simulink library "dspstat3"  (Simulink 8.0)
settings: Solver=ode45  SolverMode=SingleTasking  StartTime=0.0  StopTime=10.0  RelTol=1e-3
values from neighbouring files (symbols this model uses):
  D = D + B    [rebuffer_delay.m]
undefined symbols (not defined in the file or in its folder): Floor, Rows
libraries: dspsigattribs x3, dspsigops x1, dspindex x1, dspobslib x1, dspstat3 x1
settings Model: RequirementInfo=9  Creator=szlotkin  LastModifiedBy=lij  CovMetricSettings=d  ExtModeAutoUpdateStatusClock=off

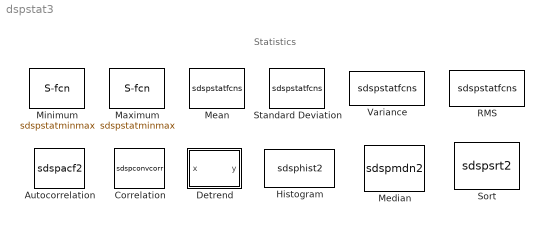
== system dspstat3 ==
  note: Statistics
  Autocorrelation : S-Function  DialogController=dspDDGCreate  DialogControllerArgs=DataTag0  FunctionName=sdspacf2  Parameters=AllPositiveLags,maxlag,bias,domain,outputMin,outputMax,dtInfo.prodOutputMode,dtInfo.prodOutputWordLength,dtInfo.prodOutputFracLength,dtInfo.accumMode,dtInfo.accumWordLength,dtInfo.accumFracLength,dtInfo.outputMode,dtInfo.outputWordLength,dtInfo.outputFracLength,dtInfo.roundingMode,dtInfo.overflowMode  EnableBusSupport=off  mask(Autocorrelation){AllPositiveLags=on, maxlag=1, bias=None, domain=Time, additionalParams=off, allowOverrides=on, outputMode=Same as accumulator, outputWordLength=16, outputFracLength=15, outputDataTypeStr=Inherit: Same as accumulator, outputLastDataTypeStr=Inherit: Same as accumulator, outputMin=[], outputMax=[], accumMode=Inherit via internal rule, accumWordLength=32, accumFracLength=30, accumDataTypeStr=Inherit: Inherit via internal rule, accumLastDataTypeStr=Inherit: Inherit via internal rule, prodOutputMode=Inherit via internal rule, prodOutputWordLength=32, prodOutputFracLength=30, prodOutputDataTypeStr=Inherit: Inherit via internal rule, prodOutputLastDataTypeStr=Inherit: Inherit via internal rule, roundingMode=Floor, overflowMode=off, LockScale=off}
      mask prompts: AllPositiveLags "Compute all non-negative lags"; maxlag "Maximum non-negative lag (less than input length):"; bias "Scaling:"; domain "Computation domain:"; additionalParams "--------------- Show additional parameters ---------------"; allowOverrides "Allow overrides from DSP Fixed-Point Attributes blocks"; outputMode "Fixed-point output attributes:"; outputWordLength "Output word length:"; outputFracLength "Output fraction length:"; outputDataTypeStr "Output data type string:"; outputLastDataTypeStr "Last output data type string:"; outputMin "Output minimum:"; outputMax "Output maximum:"; accumMode "Fixed-point accumulator attributes:"; accumWordLength "Accumulator word length:"; accumFracLength "Accumulator fraction length:"; accumDataTypeStr "Accum data type string:"; accumLastDataTypeStr "Last accum data type string:"; prodOutputMode "Fixed-point product output attributes:"; prodOutputWordLength "Product output word length:"; prodOutputFracLength "Product output fraction length:"; prodOutputDataTypeStr "ProdOutput data type string:"; prodOutputLastDataTypeStr "Last prodOutput data type string:"; roundingMode "Round integer calculations toward:"; overflowMode "Saturate on integer overflow"; LockScale "Lock scaling"
      mask help: Compute the autocorrelation along the first dimension of an N-D input array.
      mask init:
      | blkh   = gcbh;
      | dtRows = dspblkGetAutocorrelationDTRowInfo();
      | dtInfo = dspGetUDTFixptDataTypeInfo(blkh, dtRows, true);
      mask Help: eval('blocksethelp');
      mask StyleString: checkbox,edit,popup(None|Biased|Unbiased|Unity at zero-lag),popup(Time|Frequency),checkbox,checkbox,popup(Same as accumulator|Same as product output|Same as input|Binary point scaling|Slope and bias scaling|User-defined),edit,edit,unidt({a=10|12|13|}{i=Inherit: Same as input|Inherit: Same as product output|Inherit: Same as accumulator}{s=UDTBinaryPointMode}{g=UDTInheritSign}),edit,min,max,popup(Inherit via internal rule|Same as product output|Same as input|Binary point scaling|Slope and bias scaling|User-defined),edit,edit,unidt({a=17|||}{i=Inherit: Inherit via internal rule|Inherit: Same as input|Inherit: Same as product output}{s=UDTBinaryPointMode}{g=UDTInheritSign}),edit,popup(Inherit via internal rule|Same as input|Binary point scaling|Slope and bias scaling|User-defined),edit,edit,unidt({a=22|||}{i=Inherit: Inherit via internal rule|Inherit: Same as input}{s=UDTBinaryPointMode}{g=UDTInheritSign}),edit,popup(Ceiling|Convergent|Floor|Nearest|Round|Simplest|Zero),checkbox,checkbox
      mask Display: disp('ACF')
  Correlation : S-Function  DialogController=dspDDGCreate  DialogControllerArgs=DataTag1  FunctionName=sdspconvcorr  Parameters=domain,1,outputMin,outputMax,dtInfo.prodOutputMode,dtInfo.prodOutputWordLength,dtInfo.prodOutputFracLength,dtInfo.accumMode,dtInfo.accumWordLength,dtInfo.accumFracLength,dtInfo.outputMode,dtInfo.outputWordLength,dtInfo.outputFracLength,dtInfo.roundingMode,dtInfo.overflowMode  EnableBusSupport=off  mask(Correlation){domain=Time, additionalParams=off, allowOverrides=on, outputMode=Same as accumulator, outputWordLength=16, outputFracLength=15, outputDataTypeStr=Inherit: Same as accumulator, outputLastDataTypeStr=Inherit: Same as accumulator, outputMin=[], outputMax=[], accumMode=Inherit via internal rule, accumWordLength=32, accumFracLength=30, accumDataTypeStr=Inherit: Inherit via internal rule, accumLastDataTypeStr=Inherit: Inherit via internal rule, prodOutputMode=Inherit via internal rule, prodOutputWordLength=32, prodOutputFracLength=30, prodOutputDataTypeStr=Inherit: Inherit via internal rule, prodOutputLastDataTypeStr=Inherit: Inherit via internal rule, roundingMode=Floor, overflowMode=off, LockScale=off}
      mask prompts: domain "Computation domain:"; additionalParams "------- Show additional parameters -------"; allowOverrides "Allow overrides from DSP Fixed-Point Attributes blocks"; outputMode "Fixed-point output attributes:"; outputWordLength "Output word length:"; outputFracLength "Output fraction length:"; outputDataTypeStr "Output data type string:"; outputLastDataTypeStr "Last output data type string:"; outputMin "Output minimum:"; outputMax "Output maximum:"; accumMode "Fixed-point accumulator attributes:"; accumWordLength "Accumulator word length:"; accumFracLength "Accumulator fraction length:"; accumDataTypeStr "Accum data type string:"; accumLastDataTypeStr "Last accum data type string:"; prodOutputMode "Fixed-point product output attributes:"; prodOutputWordLength "Product output word length:"; prodOutputFracLength "Product output fraction length:"; prodOutputDataTypeStr "ProdOutput data type string:"; prodOutputLastDataTypeStr "Last prodOutput data type string:"; roundingMode "Round integer calculations toward:"; overflowMode "Saturate on integer overflow"; LockScale "Lock scaling"
      mask help: Correlate two inputs in the time or frequency domain. To allow the block to compute the correlation in the domain that minimizes the number of computations, set the 'Computation domain' parameter to 'Fastest'. To minimize memory usage, set the 'Computation domain' parameter to 'Time'.
      mask init:
      | blkh   = gcbh;
      | dtRows = dspblkGetCorrelationDTRowInfo();
      | dtInfo = dspGetUDTFixptDataTypeInfo(blkh, dtRows, true);
      mask Help: eval('blocksethelp');
      mask StyleString: popup(Time|Frequency|Fastest),checkbox,checkbox,popup(Same as accumulator|Same as product output|Same as first input|Binary point scaling|Slope and bias scaling|User-defined),edit,edit,unidt({a=7|9|10|}{i=Inherit: Same as first input|Inherit: Same as product output|Inherit: Same as accumulator}{s=UDTBinaryPointMode}{g=UDTInheritSign}),edit,min,max,popup(Inherit via internal rule|Same as product output|Same as first input|Binary point scaling|Slope and bias scaling|User-defined),edit,edit,unidt({a=14|||}{i=Inherit: Inherit via internal rule|Inherit: Same as first input|Inherit: Same as product output}{s=UDTBinaryPointMode}{g=UDTInheritSign}),edit,popup(Inherit via internal rule|Same as first input|Binary point scaling|Slope and bias scaling|User-defined),edit,edit,unidt({a=19|||}{i=Inherit: Inherit via internal rule|Inherit: Same as first input}{s=UDTBinaryPointMode}{g=UDTInheritSign}),edit,popup(Ceiling|Convergent|Floor|Nearest|Round|Simplest|Zero),checkbox,checkbox
      mask Display: disp('XCORR')
  Detrend : Subsystem
      mask Type: Detrend
      mask Description: Remove linear trend from vector input.
      mask Help: eval('blocksethelp');
      mask Display: plot(0,0,100,100,[12 20 24 32 38 44 49 54 67 69 71 78 81 89],[56 76 60 79 75 83 80 87 65 76 84 86 91 89],[],[],[],[],[],[],[12 20 24 32 38 44 49 54 67 69 71 78 81 89],[12 31 13 31 27 34 30 36 13 23 30 31 34 32],[4 96],[61 90],[47 47 42 47 52],[64 44 50 44 50],[4 96],[23 23])
  Histogram : S-Function  DialogController=dvDDGCreate  DialogControllerArgs=DataTag4  FunctionName=sdsphist2  Parameters=umin,umax,nbins,normalized,run,reset,trigtype,operateOver,1,1,0,dtInfo.prodOutputMode,dtInfo.prodOutputWordLength,dtInfo.prodOutputFracLength,dtInfo.accumMode,dtInfo.accumWordLength,dtInfo.accumFracLength,dtInfo.roundingMode,dtInfo.overflowMode  EnableBusSupport=off  mask(Histogram){umin=0, umax=10, nbins=11, normalized=off, run=off, reset=on, trigtype=Non-zero sample, operateOver=Each column, Dimension=1, colComp=on, additionalParams=off, allowOverrides=on, accumMode=Same as input, accumWordLength=32, accumFracLength=30, accumDataTypeStr=Inherit: Same as input, accumLastDataTypeStr=Inherit: Same as input, prodOutputMode=Same as input, prodOutputWordLength=32, prodOutputFracLength=30, prodOutputDataTypeStr=Inherit: Same as input, prodOutputLastDataTypeStr=Inherit: Same as input, roundingMode=Floor, overflowMode=off, LockScale=off}
      mask prompts: umin "Lower limit of histogram:"; umax "Upper limit of histogram:"; nbins "Number of bins:"; run "Running histogram"; reset "Reset port"; trigtype "Trigger type:"; operateOver "Find the histogram over"; colComp "Column compatibility"; additionalParams "--------------- Show additional parameters ---------------"; allowOverrides "Allow overrides from DSP Attributes blocks"; accumMode "Fixed-point accumulator attributes"; accumWordLength "Accumulator word length:"; accumFracLength "Accumulator fraction length:"; accumDataTypeStr "Accum data type string:"; accumLastDataTypeStr "Last accum data type string:"; prodOutputMode "Fixed-point product output attributes:"; prodOutputWordLength "Product output word length:"; prodOutputFracLength "Product output fraction length:"; prodOutputDataTypeStr "ProdOutput data type string:"; prodOutputLastDataTypeStr "Last prodOutput data type string:"; roundingMode "Round integer calculations toward:"; overflowMode "Saturate on integer overflow"; LockScale "Lock scaling"
      mask help: Generate a histogram of the elements in the specified dimension of the input or across time (running histogram).
      mask init:
      | blkh     = gcbh;
      | dspSetFrameUpgradeParameter(blkh, 'operateOver', 'Inherited (this choice will be removed - see release notes)');
      | trigtype = trigtype-1;
      | dtRows   = dspblkGetHistogramDTRowInfo();
      | dtInfo   = dspGetUDTFixptDataTypeInfo(blkh, dtRows, true);
      mask Help: eval('blocksethelp');
      mask StyleString: edit,edit,edit,checkbox,checkbox,checkbox,popup(None|Rising edge|Falling edge|Either edge|Non-zero sample),popup(Entire input|Each column|Inherited (this choice will be removed - see release notes)),edit,checkbox,checkbox,checkbox,popup(Same as product output|Same as input|Binary point scaling|Slope and bias scaling|User-defined),edit,edit,unidt({a=16|||}{i=Inherit: Same as input|Inherit: Same as product output}{s=UDTBinaryPointMode}{g=UDTInheritSign}),edit,popup(Same as input|Binary point scaling|Slope and bias scaling|User-defined),edit,edit,unidt({a=21|||}{i=Inherit: Same as input}{s=UDTBinaryPointMode}{g=UDTInheritSign}),edit,popup(Ceiling|Convergent|Floor|Nearest|Round|Simplest|Zero),checkbox,checkbox
      mask Display:
      | [s,x,y] = dspblkhist2('icon');
      | plot(x,y);
      | port_label('input',s.i1,s.i1s);
      | port_label('input',s.i2,s.i2s);
  Maximum : S-Function  DialogController=dvDDGCreate  DialogControllerArgs=DataTag6  FunctionName=sdspstatminmax  Parameters=statfcn,fcn,reset,InputProcessing,opOvr,colComp,idxBase,Dimension,roiEnable,roiType,roiPortion,roiOutput,roiFlag,dtInfo.prodOutputMode,dtInfo.prodOutputWordLength,dtInfo.prodOutputFracLength,dtInfo.accumMode,dtInfo.accumWordLength,dtInfo.accumFracLength,dtInfo.roundingMode,dtInfo.overflowMode  EnableBusSupport=off  mask(Maximum){fcn=Value and Index, reset=None, InputProcessing=Columns as channels (frame based), indexBase=One, operateOver=Each column, Dimension=1, colComp=on, operation=maximum, roiEnable=off, roiType=Rectangles, roiPortion=Entire ROI, roiOutput=Individual statistics for each ROI, roiFlag=off, additionalParams=off, allowOverrides=on, accumMode=Same as product output, accumWordLength=32, accumFracLength=30, accumDataTypeStr=Inherit: Same as product output, accumLastDataTypeStr=Inherit: Same as product output, prodOutputMode=Same as input, prodOutputWordLength=32, prodOutputFracLength=30, prodOutputDataTypeStr=Inherit: Same as input, prodOutputLastDataTypeStr=Inherit: Same as input, roundingMode=Floor, overflowMode=off, LockScale=off}
      mask prompts: fcn "Mode:"; reset "Reset port:"; InputProcessing "Input processing:"; indexBase "Index Base"; operateOver "Operate over"; colComp "Column compatibility"; roiEnable "Enable ROI processing"; roiType "ROI type:"; roiPortion "ROI portion to process:"; roiOutput "Output:"; roiFlag "Output flag indicating if ROI is completely out of image bounds"; additionalParams "--------------- Show additional parameters ---------------"; allowOverrides "Allow overrides from DSP Attributes blocks"; accumMode "Fixed-point accumulator attributes:"; accumWordLength "Accumulator word length:"; accumFracLength "Accumulator fraction length:"; accumDataTypeStr "Accum data type string:"; accumLastDataTypeStr "Last accum data type string:"; prodOutputMode "Fixed-point product output attributes:"; prodOutputWordLength "Product output word length:"; prodOutputFracLength "Product output fraction length:"; prodOutputDataTypeStr "ProdOutput data type string:"; prodOutputLastDataTypeStr "Last prodOutput data type string:"; roundingMode "Round integer calculations toward:"; overflowMode "Saturate on integer overflow"; LockScale "Lock scaling"
      mask help: Compute the maximum value along the specified dimension of the input or across time (running maximum).
      mask init:
      | blkh = gcbh;
      | dspSetFrameUpgradeParameter(blkh, 'InputProcessing', 'Inherited (this choice will be removed - see release notes)', 'fcn', 'Running');
      | reset=reset-1;
      | statfcn=5;
      | map = [0 2 3 1];
      | fcn = map(fcn);
      | dtRows = dspblkGetMaximumDTRowInfo();
      | dtInfo = dspGetUDTFixptDataTypeInfo(blkh, dtRows, true);
      | map = [1 0];
      | idxBase = map(indexBase);
      | map = [2 0 1 3];
      | opOvr = map(operateOver);
      mask Help: eval('blocksethelp');
      mask StyleString: popup(Value and Index|Value|Index|Running),popup(None|Rising edge|Falling edge|Either edge|Non-zero sample),popup(Columns as channels (frame based)|Elements as channels (sample based)|Inherited (this choice will be removed - see release notes)),popup(Zero|One),popup(Entire input|Each row|Each column|Specified dimension),edit,checkbox,popup(maximum),checkbox,popup(Rectangles|Lines|Label matrix|Binary mask),popup(Entire ROI|ROI perimeter),popup(Individual statistics for each ROI|Single statistic for all ROIs),checkbox,checkbox,checkbox,popup(Same as product output|Same as input|Binary point scaling|Slope and bias scaling|User-defined),edit,edit,unidt({a=19|||}{i=Inherit: Same as input|Inherit: Same as product output}{s=UDTBinaryPointMode}{g=UDTInheritSign}),edit,popup(Same as input|Binary point scaling|Slope and bias scaling|User-defined),edit,edit,unidt({a=24|||}{i=Inherit: Same as input}{s=UDTBinaryPointMode}{g=UDTInheritSign}),edit,popup(Ceiling|Convergent|Floor|Nearest|Round|Simplest|Zero),checkbox,checkbox
      mask Display:
      | [s, x, y] = dspblkminmax('max');
      | plot(x,y);
      | port_label('input',s.i1,s.i1s);
      | port_label('input',s.i2,s.i2s);
      | port_label('input',s.i3,s.i3s);
      | port_label('output',s.o1,s.o1s);
      | port_label('output',s.o2,s.o2s);
      | port_label('output',s.o3,s.o3s);
  Mean : S-Function  DialogController=dvDDGCreate  DialogControllerArgs=DataTag8  FunctionName=sdspstatfcns  Parameters=fcn,run,reset,InputProcessing,directionMode,treatSBRowAsCol,dimension,roiEnable,roiType,roiPortion,roiOutput,roiFlag,outputMin,outputMax,0,16,0,dtInfo.accumMode,dtInfo.accumWordLength,dtInfo.accumFracLength,0,2,0,dtInfo.outputMode,dtInfo.outputWordLength,dtInfo.outputFracLength,dtInfo.roundingMode,dtInfo.overflowMode  EnableBusSupport=off  mask(Mean){run=off, reset_popup=None, InputProcessing=Columns as channels (frame based), directionMode=Each column, dimension=1, treatSBRowAsCol=on, roiEnable=off, roiType=Rectangles, roiPortion=Entire ROI, roiOutput=Individual statistics for each ROI, roiFlag=off, additionalParams=off, allowOverrides=on, outputMode=Same as accumulator, outputWordLength=32, outputFracLength=30, outputDataTypeStr=Inherit: Same as accumulator, outputLastDataTypeStr=Inherit: Same as accumulator, outputMin=[], outputMax=[], accumMode=Same as input, accumWordLength=32, accumFracLength=30, accumDataTypeStr=Inherit: Same as input, accumLastDataTypeStr=Inherit: Same as input, roundingMode=Floor, overflowMode=off, LockScale=off}
      mask prompts: run "Running mean"; reset_popup "Reset port"; InputProcessing "Input processing:"; directionMode "Find the mean value over:"; treatSBRowAsCol "Treat sample-based row input as a column"; roiEnable "Enable ROI processing"; roiType "ROI type:"; roiPortion "ROI portion to process:"; roiOutput "Output:"; roiFlag "Output flag indicating if ROI is completely out of image bounds"; additionalParams "--------------- Show additional parameters ---------------"; allowOverrides "Allow overrides from DSP Attributes blocks"; outputMode "Fixed-point output attributes:"; outputWordLength "Output word length:"; outputFracLength "Output fraction length:"; outputDataTypeStr "Output data type string:"; outputLastDataTypeStr "Last output data type string:"; outputMin "Output minimum:"; outputMax "Output maximum:"; accumMode "Fixed-point accumulator attributes"; accumWordLength "Accumulator word length:"; accumFracLength "Accumulator fraction length:"; accumDataTypeStr "Accum data type string:"; accumLastDataTypeStr "Last accum data type string:"; roundingMode "Round integer calculations toward:"; overflowMode "Saturate on integer overflow"; LockScale "Lock scaling"
      mask help: Compute the mean value along the specified dimension of the input or across time (running mean).
      mask init:
      | blkh = gcbh;
      | dspSetFrameUpgradeParameter(blkh, 'InputProcessing', 'Inherited (this choice will be removed - see release notes)', 'run', 'on');
      | reset=reset_popup-1;
      | fcn=3;
      | dtRows = dspblkGetMeanDTRowInfo();
      | dtInfo = dspGetUDTFixptDataTypeInfo(blkh, dtRows, true);
      mask Help: eval('blocksethelp');
      mask StyleString: checkbox,popup(None|Rising edge|Falling edge|Either edge|Non-zero sample),popup(Columns as channels (frame based)|Elements as channels (sample based)|Inherited (this choice will be removed - see release notes)),popup(Entire input|Each row|Each column|Specified dimension),edit,checkbox,checkbox,popup(Rectangles|Lines|Label matrix|Binary mask),popup(Entire ROI|ROI perimeter),popup(Individual statistics for each ROI|Single statistic for all ROIs),checkbox,checkbox,checkbox,popup(Same as accumulator|Same as input|Binary point scaling|Slope and bias scaling|User-defined),edit,edit,unidt({a=17|19|20|}{i=Inherit: Same as input|Inherit: Same as accumulator}{s=UDTBinaryPointMode}{g=UDTInheritSign}),edit,min,max,popup(Same as input|Binary point scaling|Slope and bias scaling|User-defined),edit,edit,unidt({a=24|||}{i=Inherit: Same as input}{s=UDTBinaryPointMode}{g=UDTInheritSign}),edit,popup(Ceiling|Convergent|Floor|Nearest|Round|Simplest|Zero),checkbox,checkbox
      mask Display:
      | [s,x,y] = dspblkmean2;
      | plot(x,y);
      | port_label('input',s.i1,s.i1s);
      | port_label('input',s.i2,s.i2s);
      | port_label('input',s.i3,s.i3s);
      | 
      | port_label('output',s.o1,s.o1s);
      | port_label('output',s.o2,s.o2s);
  Median : S-Function  DialogController=dvDDGCreate  DialogControllerArgs=DataTag9  FunctionName=sdspmdn2  Parameters=sortAlg,directionMode,treatSBRowAsCol,dimension,outputMin,outputMax,dtInfo.prodOutputMode,dtInfo.prodOutputWordLength,dtInfo.prodOutputFracLength,dtInfo.accumMode,dtInfo.accumWordLength,dtInfo.accumFracLength,dtInfo.outputMode,dtInfo.outputWordLength,dtInfo.outputFracLength,dtInfo.roundingMode,dtInfo.overflowMode  EnableBusSupport=off  mask(Median){sortAlg=Quick sort, directionMode=Each column, dimension=1, treatSBRowAsCol=on, additionalParams=off, allowOverrides=off, outputMode=Same as accumulator, outputWordLength=16, outputFracLength=15, outputDataTypeStr=Inherit: Same as accumulator, outputLastDataTypeStr=Inherit: Same as accumulator, outputMin=[], outputMax=[], accumMode=Same as product output, accumWordLength=32, accumFracLength=30, accumDataTypeStr=Inherit: Same as product output, accumLastDataTypeStr=Inherit: Same as product output, prodOutputMode=Same as input, prodOutputWordLength=32, prodOutputFracLength=30, prodOutputDataTypeStr=Inherit: Same as input, prodOutputLastDataTypeStr=Inherit: Same as input, roundingMode=Floor, overflowMode=off, LockScale=off}
      mask prompts: sortAlg "Sort algorithm:"; directionMode "Find the median value over:"; treatSBRowAsCol "Treat sample-based row input as a column"; additionalParams "--------------- Show additional parameters ---------------"; allowOverrides "Allow overrides from DSP Attributes blocks"; outputMode "Fixed-point output attributes:"; outputWordLength "Output word length:"; outputFracLength "Output fraction length:"; outputDataTypeStr "Output data type string:"; outputLastDataTypeStr "Last output data type string:"; outputMin "Output minimum:"; outputMax "Output maximum:"; accumMode "Fixed-point accumulator attributes"; accumWordLength "Accumulator word length:"; accumFracLength "Accumulator fraction length:"; accumDataTypeStr "Accum data type string:"; accumLastDataTypeStr "Last accum data type string:"; prodOutputMode "Fixed-point product output attributes:"; prodOutputWordLength "Product output word length:"; prodOutputFracLength "Product output fraction length:"; prodOutputDataTypeStr "ProdOutput data type string:"; prodOutputLastDataTypeStr "Last prodOutput data type string:"; roundingMode "Round integer calculations toward:"; overflowMode "Saturate on integer overflow"; LockScale "Lock scaling"
      mask help:
      | Compute the median value along the specified dimension of the input or across time (running median).
      |
      | The 'Product output' and 'Accumulator' parameters apply only for complex fixed-point inputs.
      mask init:
      | blkh   = gcbh;
      | dtRows = dspblkGetMedianDTRowInfo();
      | dtInfo = dspGetUDTFixptDataTypeInfo(blkh, dtRows, true);
      mask Help: eval('blocksethelp');
      mask StyleString: popup(Quick sort|Insertion sort),popup(Entire input|Each row|Each column|Specified dimension),edit,checkbox,checkbox,checkbox,popup(Same as accumulator|Same as product output|Same as input|Binary point scaling|Slope and bias scaling|User-defined),edit,edit,unidt({a=10|12|13|}{i=Inherit: Same as input|Inherit: Same as product output|Inherit: Same as accumulator}{s=UDTBinaryPointMode}{g=UDTInheritSign}),edit,min,max,popup(Same as product output|Same as input|Binary point scaling|Slope and bias scaling|User-defined),edit,edit,unidt({a=17|||}{i=Inherit: Same as input|Inherit: Same as product output}{s=UDTBinaryPointMode}{g=UDTInheritSign}),edit,popup(Same as input|Binary point scaling|Slope and bias scaling|User-defined),edit,edit,unidt({a=22|||}{i=Inherit: Same as input}{s=UDTBinaryPointMode}{g=UDTInheritSign}),edit,popup(Ceiling|Convergent|Floor|Nearest|Round|Simplest|Zero),checkbox,checkbox
      mask Display:
      | [x, y] = dspblkmedian();
      | plot(x,y);
  Minimum : S-Function  DialogController=dvDDGCreate  DialogControllerArgs=DataTag11  FunctionName=sdspstatminmax  Parameters=statfcn,fcn,reset,InputProcessing,opOvr,colComp,idxBase,Dimension,roiEnable,roiType,roiPortion,roiOutput,roiFlag,dtInfo.prodOutputMode,dtInfo.prodOutputWordLength,dtInfo.prodOutputFracLength,dtInfo.accumMode,dtInfo.accumWordLength,dtInfo.accumFracLength,dtInfo.roundingMode,dtInfo.overflowMode  EnableBusSupport=off  mask(Minimum){fcn=Value and Index, reset=None, InputProcessing=Columns as channels (frame based), indexBase=One, operateOver=Each column, Dimension=1, colComp=on, operation=minimum, roiEnable=off, roiType=Rectangles, roiPortion=Entire ROI, roiOutput=Individual statistics for each ROI, roiFlag=off, additionalParams=off, allowOverrides=on, accumMode=Same as input, accumWordLength=32, accumFracLength=30, accumDataTypeStr=Inherit: Same as input, accumLastDataTypeStr=Inherit: Same as input, prodOutputMode=Same as input, prodOutputWordLength=32, prodOutputFracLength=30, prodOutputDataTypeStr=Inherit: Same as input, prodOutputLastDataTypeStr=Inherit: Same as input, roundingMode=Floor, overflowMode=off, LockScale=off}
      mask prompts: fcn "Mode:"; reset "Reset port"; InputProcessing "Input processing:"; indexBase "Index base"; operateOver "Operate over"; colComp "Column compatibility"; roiEnable "Enable ROI processing"; roiType "ROI type:"; roiPortion "ROI portion to process:"; roiOutput "Output:"; roiFlag "Output flag indicating if ROI is completely out of image bounds"; additionalParams "--------------- Show additional parameters ---------------"; allowOverrides "Allow overrides from DSP Attributes blocks"; accumMode "Fixed-point accumulator attributes:"; accumWordLength "Accumulator word length:"; accumFracLength "Accumulator fraction length:"; accumDataTypeStr "Accum data type string:"; accumLastDataTypeStr "Last accum data type string:"; prodOutputMode "Fixed-point product output attributes:"; prodOutputWordLength "Product output word length:"; prodOutputFracLength "Product output fraction length:"; prodOutputDataTypeStr "ProdOutput data type string:"; prodOutputLastDataTypeStr "Last prodOutput data type string:"; roundingMode "Round integer calculations toward:"; overflowMode "Saturate on integer overflow"; LockScale "Lock scaling"
      mask help: Compute the minimum value along the specified dimension of the input or across time (running minimum).
      mask init:
      | blkh = gcbh;
      | dspSetFrameUpgradeParameter(blkh, 'InputProcessing', 'Inherited (this choice will be removed - see release notes)', 'fcn', 'Running');
      | reset=reset-1;
      | statfcn=4;
      | map = [0 2 3 1];
      | fcn = map(fcn);
      | dtRows = dspblkGetMinimumDTRowInfo();
      | dtInfo = dspGetUDTFixptDataTypeInfo(blkh, dtRows, true);
      | map = [1 0];
      | idxBase = map(indexBase);
      | map = [2 0 1 3];
      | opOvr = map(operateOver);
      mask Help: eval('blocksethelp');
      mask StyleString: popup(Value and Index|Value|Index|Running),popup(None|Rising edge|Falling edge|Either edge|Non-zero sample),popup(Columns as channels (frame based)|Elements as channels (sample based)|Inherited (this choice will be removed - see release notes)),popup(Zero|One),popup(Entire input|Each row|Each column|Specified dimension),edit,checkbox,popup(minimum),checkbox,popup(Rectangles|Lines|Label matrix|Binary mask),popup(Entire ROI|ROI perimeter),popup(Individual statistics for each ROI|Single statistic for all ROIs),checkbox,checkbox,checkbox,popup(Same as product output|Same as input|Binary point scaling|Slope and bias scaling|User-defined),edit,edit,unidt({a=19|||}{i=Inherit: Same as input|Inherit: Same as product output}{s=UDTBinaryPointMode}{g=UDTInheritSign}),edit,popup(Same as input|Binary point scaling|Slope and bias scaling|User-defined),edit,edit,unidt({a=24|||}{i=Inherit: Same as input}{s=UDTBinaryPointMode}{g=UDTInheritSign}),edit,popup(Ceiling|Convergent|Floor|Nearest|Round|Simplest|Zero),checkbox,checkbox
      mask Display:
      | [s, x, y] = dspblkminmax('min');
      | plot(x,y);
      | port_label('input',s.i1,s.i1s);
      | port_label('input',s.i2,s.i2s);
      | port_label('input',s.i3,s.i3s);
      | port_label('output',s.o1,s.o1s);
      | port_label('output',s.o2,s.o2s);
      | port_label('output',s.o3,s.o3s);
  RMS : S-Function  DialogController=dspDDGCreate  DialogControllerArgs=DataTag13  FunctionName=sdspstatfcns  Parameters=fcn,run,reset,InputProcessing,directionMode,treatSBRowAsCol,dimension  EnableBusSupport=off  mask(RMS){run=off, reset_popup=None, InputProcessing=Columns as channels (frame based), directionMode=Each column, dimension=1, treatSBRowAsCol=on}
      mask prompts: run "Running RMS"; reset_popup "Reset port"; InputProcessing "Input processing:"; directionMode "Find the RMS value over:"; treatSBRowAsCol "Treat sample-based row input as a column"
      mask help: Compute the root-mean-square (RMS) along the specified dimension of the input or across time (running RMS).
      mask init:
      | dspSetFrameUpgradeParameter(gcbh, 'InputProcessing', 'Inherited (this choice will be removed - see release notes)', 'run', 'on');
      | fcn=2;
      | reset=reset_popup-1;
      mask Help: eval('blocksethelp');
      mask StyleString: checkbox,popup(None|Rising edge|Falling edge|Either edge|Non-zero sample),popup(Columns as channels (frame based)|Elements as channels (sample based)|Inherited (this choice will be removed - see release notes)),popup(Entire input|Each row|Each column|Specified dimension),edit,checkbox
      mask Display:
      | [s,x] = dspblkrms2;
      | disp(x);
      | port_label('input',s.i1,s.i1s);
      | port_label('input',s.i2,s.i2s);
  Sort : S-Function  DialogController=dspDDGCreate  DialogControllerArgs=DataTag14  FunctionName=sdspsrt2  Parameters=dir,otype,sortAlg,dtInfo.prodOutputMode,dtInfo.prodOutputWordLength,dtInfo.prodOutputFracLength,dtInfo.accumMode,dtInfo.accumWordLength,dtInfo.accumFracLength,dtInfo.roundingMode,dtInfo.overflowMode  EnableBusSupport=off  mask(Sort){otype=Value and Index, dir=Ascending, sortAlg=Quick sort, additionalParams=off, allowOverrides=on, accumMode=Same as product output, accumWordLength=32, accumFracLength=30, accumDataTypeStr=Inherit: Same as product output, accumLastDataTypeStr=Inherit: Same as product output, prodOutputMode=Same as input, prodOutputWordLength=32, prodOutputFracLength=30, prodOutputDataTypeStr=Inherit: Same as input, prodOutputLastDataTypeStr=Inherit: Same as input, roundingMode=Floor, overflowMode=off, LockScale=off}
      mask prompts: otype "Mode:"; dir "Sort order:"; sortAlg "Sort algorithm:"; additionalParams "--------------- Show additional parameters ---------------"; allowOverrides "Allow overrides from DSP Attributes blocks"; accumMode "Fixed-point accumulator attributes"; accumWordLength "Accumulator word length:"; accumFracLength "Accumulator fraction length:"; accumDataTypeStr "Accum data type string:"; accumLastDataTypeStr "Last accum data type string:"; prodOutputMode "Fixed-point product output attributes:"; prodOutputWordLength "Product output word length:"; prodOutputFracLength "Product output fraction length:"; prodOutputDataTypeStr "ProdOutput data type string:"; prodOutputLastDataTypeStr "Last prodOutput data type string:"; roundingMode "Round integer calculations toward:"; overflowMode "Saturate on integer overflow"; LockScale "Lock scaling"
      mask help:
      | Value and/or index of sorted elements in vector or matrix.  For matrix inputs, the elements are sorted columnwise.
      |
      | The 'Product output' and 'Accumulator' parameters apply only for complex fixed-point inputs.
      mask init:
      | blkh   = gcbh;
      | dtRows = dspblkGetSortDTRowInfo();
      | dtInfo = dspGetUDTFixptDataTypeInfo(blkh, dtRows, true);
      mask Help: eval('blocksethelp');
      mask StyleString: popup(Value and Index|Value|Index),popup(Ascending|Descending),popup(Quick sort|Insertion sort),checkbox,checkbox,popup(Same as product output|Same as input|Binary point scaling|Slope and bias scaling|User-defined),edit,edit,unidt({a=9|||}{i=Inherit: Same as input|Inherit: Same as product output}{s=UDTBinaryPointMode}{g=UDTInheritSign}),edit,popup(Same as input|Binary point scaling|Slope and bias scaling|User-defined),edit,edit,unidt({a=14|||}{i=Inherit: Same as input}{s=UDTBinaryPointMode}{g=UDTInheritSign}),edit,popup(Ceiling|Convergent|Floor|Nearest|Round|Simplest|Zero),checkbox,checkbox
      mask Display:
      | [s,x,y] = dspblksort('icon',dir,otype);
      | plot(x,y);
      | port_label('input',s.i1,s.i1s);
      | port_label('input',s.i2,s.i2s);
      | port_label('output',s.o1,s.o1s);
      | port_label('output',s.o2,s.o2s);
  Standard Deviation : S-Function  DialogController=dvDDGCreate  DialogControllerArgs=DataTag16  FunctionName=sdspstatfcns  Parameters=fcn,run,reset,InputProcessing,directionMode,treatSBRowAsCol,dimension,roiEnable,roiType,roiPortion,roiOutput,roiFlag  EnableBusSupport=off  mask(Standard Deviation){run=off, reset_popup=None, InputProcessing=Columns as channels (frame based), directionMode=Each column, dimension=1, treatSBRowAsCol=on, roiEnable=off, roiType=Rectangles, roiPortion=Entire ROI, roiOutput=Individual statistics for each ROI, roiFlag=off}
      mask prompts: run "Running standard deviation"; reset_popup "Reset port"; InputProcessing "Input processing:"; directionMode "Find the standard deviation value over:"; treatSBRowAsCol "Treat sample-based row input as a column"; roiEnable "Enable ROI processing"; roiType "ROI type:"; roiPortion "ROI portion to process:"; roiOutput "Output:"; roiFlag "Output flag indicating if ROI is completely out of image bounds"
      mask help: Compute the standard deviation along the specified dimension of the input or across time (running standard deviation).
      mask init:
      | dspSetFrameUpgradeParameter(gcbh, 'InputProcessing', 'Inherited (this choice will be removed - see release notes)', 'run', 'on');
      | fcn=1;
      | %Set the flag to compute the standard deviation
      | reset=reset_popup-1;
      mask Help: eval('blocksethelp');
      mask StyleString: checkbox,popup(None|Rising edge|Falling edge|Either edge|Non-zero sample),popup(Columns as channels (frame based)|Elements as channels (sample based)|Inherited (this choice will be removed - see release notes)),popup(Entire input|Each row|Each column|Specified dimension),edit,checkbox,checkbox,popup(Rectangles|Lines|Label matrix|Binary mask),popup(Entire ROI|ROI perimeter),popup(Individual statistics for each ROI|Single statistic for all ROIs),checkbox
      mask Display:
      | [s,x,y] = dspblkstd2;
      | plot(x,y);
      | port_label('input',s.i1,s.i1s);
      | port_label('input',s.i2,s.i2s);
      | port_label('input',s.i3,s.i3s);
      | 
      | port_label('output',s.o1,s.o1s);
      | port_label('output',s.o2,s.o2s);
  Variance : S-Function  DialogController=dvDDGCreate  DialogControllerArgs=DataTag18  FunctionName=sdspstatfcns  Parameters=fcn,run,reset,InputProcessing,directionMode,treatSBRowAsCol,dimension,roiEnable,roiType,roiPortion,roiOutput,roiFlag,[],[],dtInfo.prodOutputMode,dtInfo.prodOutputWordLength,dtInfo.prodOutputFracLength,dtInfo.accumMode,dtInfo.accumWordLength,dtInfo.accumFracLength,dtInfo.memoryMode,dtInfo.memoryWordLength,dtInfo.memoryFracLength,dtInfo.outputMode,dtInfo.outputWordLength,dtInfo.outputFracLength,dtInfo.roundingMode,dtInfo.overflowMode  EnableBusSupport=off  mask(Variance){run=off, reset_popup=None, InputProcessing=Columns as channels (frame based), directionMode=Each column, dimension=1, treatSBRowAsCol=on, roiEnable=off, roiType=Rectangles, roiPortion=Entire ROI, roiOutput=Individual statistics for each ROI, roiFlag=off, additionalParams=off, allowOverrides=on, outputMode=Same as input-squared product, outputWordLength=32, outputFracLength=30, accumMode=Same as input-squared product, accumWordLength=32, accumFracLength=30, prodOutputMode=Same as input, prodOutputWordLength=32, prodOutputFracLength=30, memoryMode=Same as input-squared product, memoryWordLength=32, memoryFracLength=30, roundingMode=Floor, overflowMode=off, LockScale=off}
      mask prompts: run "Running variance"; reset_popup "Reset port"; InputProcessing "Input processing:"; directionMode "Find the mean value over:"; treatSBRowAsCol "Treat sample-based row input as a column"; roiEnable "Enable ROI processing"; roiType "ROI type:"; roiPortion "ROI portion to process:"; roiOutput "Output:"; roiFlag "Output flag indicating if ROI is completely out of image bounds"; additionalParams "--------------- Show additional parameters ---------------"; allowOverrides "Allow overrides from DSP Attributes blocks"; outputMode "Fixed-point output attributes:"; outputWordLength "Output word length:"; outputFracLength "Output fraction length:"; accumMode "Fixed-point accumulator attributes"; accumWordLength "Accumulator word length:"; accumFracLength "Accumulator fraction length:"; prodOutputMode "Fixed-point input-squared product output attributes:"; prodOutputWordLength "Input-squared product word length:"; prodOutputFracLength "Input-squared product fraction length:"; memoryMode "Fixed-poing input-sum-squared product attributes:"; memoryWordLength "Input-sum-squared product word length:"; memoryFracLength "Input-sum-squared product fraction length:"; roundingMode "Round integer calculations toward:"; overflowMode "Saturate on integer overflow"; LockScale "Lock scaling"
      mask help: Compute the variance along the specified dimension of the input or across time (running variance).
      mask init:
      | blkh = gcbh;
      | dspSetFrameUpgradeParameter(blkh, 'InputProcessing', 'Inherited (this choice will be removed - see release notes)', 'run', 'on');
      | fcn=0; %Set the flag to compute the variance
      | reset=reset_popup-1;
      | dtInfo = dspGetFixptDataTypeInfo(blkh,31);
      mask Help: eval('blocksethelp');
      mask StyleString: checkbox,popup(None|Rising edge|Falling edge|Either edge|Non-zero sample),popup(Columns as channels (frame based)|Elements as channels (sample based)|Inherited (this choice will be removed - see release notes)),popup(Entire input|Each row|Each column|Specified dimension),edit,checkbox,checkbox,popup(Rectangles|Lines|Label matrix|Binary mask),popup(Entire ROI|ROI perimeter),popup(Individual statistics for each ROI|Single statistic for all ROIs),checkbox,checkbox,checkbox,popup(Same as accumulator|Same as input-squared product|Same as input|Binary point scaling|Slope and bias scaling|User-defined),edit,edit,popup(Same as input-squared product|Same as input|Binary point scaling|Slope and bias scaling|User-defined),edit,edit,popup(Same as input|Binary point scaling|Slope and bias scaling|User-defined),edit,edit,popup(Same as input-squared product|Binary point scaling|Slope and bias scaling),edit,edit,popup(Ceiling|Convergent|Floor|Nearest|Round|Simplest|Zero),checkbox,checkbox
      mask Display:
      | [s,x] = dspblkvar2;
      | disp(x);
      | port_label('input',s.i1,s.i1s);
      | port_label('input',s.i2,s.i2s);
      | port_label('input',s.i3,s.i3s);
      | 
      | port_label('output',s.o1,s.o1s);
      | port_label('output',s.o2,s.o2s);

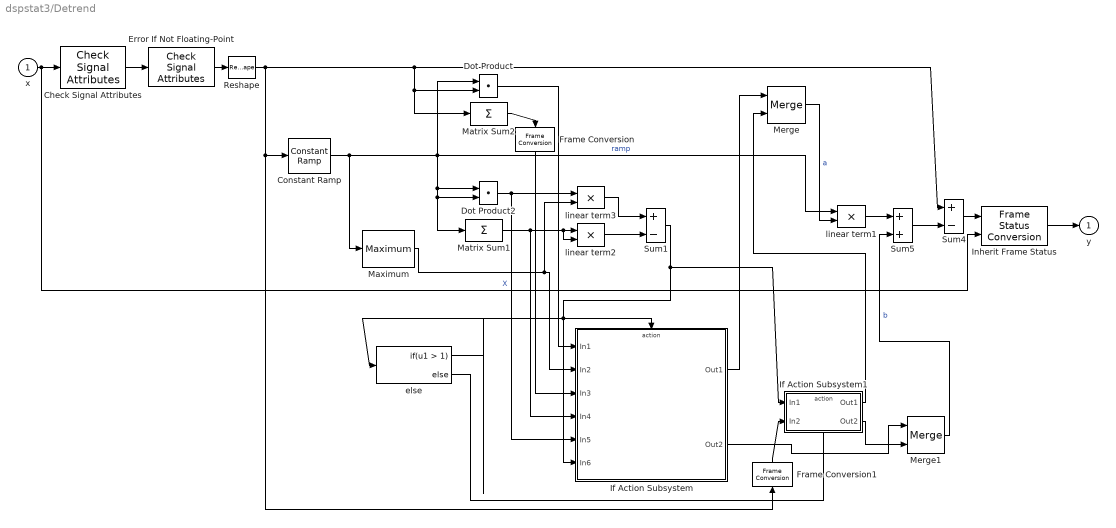
== system dspstat3/Detrend ==
  x : Inport
  Check Signal Attributes : dspsigattribs/Check Signal Attributes  SystemSampleTime=-1  SigAttribCheckMethod=Does not match attributes exactly  Complexity=Ignore  Frame=Ignore  DimsCheckMethod=Is...  Dimensions=Vector (1-D or 2-D) or scalar  DatatypeCheckMethod=Ignore  DatatypeGeneral=Boolean  DtypeFloatSpecific=Any floating-point  DtypeFixedSpecific=Any fixed-point  DtypeIntSpecific=Any integer  SampleMode=Ignore
  Constant Ramp : dspsigops/Constant Ramp  L=Rows  dim=1  Slope=1  dataType=Same as input  isSigned=on  wordLen=16  udDataType=sfix(16)  fracBitsMode=Best precision  numFracBits=15  Offset=1
  Dot Product : DotProduct  OutDataTypeStr=Inherit: Inherit via internal rule
  Dot Product2 : DotProduct  OutDataTypeStr=Inherit: Inherit via internal rule
  Error If Not Floating-Point : dspsigattribs/Check Signal Attributes  SystemSampleTime=-1  SigAttribCheckMethod=Does not match attributes exactly  Complexity=Ignore  Frame=Ignore  DimsCheckMethod=Ignore  Dimensions=1-D  DatatypeCheckMethod=Is...  DatatypeGeneral=Floating-point  DtypeFloatSpecific=Any floating-point  DtypeFixedSpecific=Any fixed-point  DtypeIntSpecific=Any integer  SampleMode=Ignore
  Frame Conversion : FrameConversion  OutFrame=Sample-based
  Frame Conversion1 : FrameConversion  OutFrame=Sample-based
  If Action Subsystem : Subsystem  TreatAsAtomicUnit=on
  If Action Subsystem1 : Subsystem  TreatAsAtomicUnit=on
  Inherit Frame Status : dspobslib/Frame Status Conversion  SystemSampleTime=-1  growRefPort=on  outframe=Frame-based
  Matrix Sum1 : Sum  Inputs=+  CollapseMode=Specified dimension  OutDataTypeStr=Inherit: Same as first input
  Matrix Sum2 : Sum  Inputs=+  CollapseMode=Specified dimension  OutDataTypeStr=Inherit: Same as first input
  Maximum : dspstat3/Maximum  fcn=Value  reset=None  InputProcessing=Columns as channels (frame based)  indexBase=One  operateOver=Each column  Dimension=1  colComp=on  operation=maximum  roiEnable=off  roiType=Rectangles  roiPortion=Entire ROI  roiOutput=Individual statistics for each ROI  roiFlag=off  accumDataTypeStr=Inherit: Same as product output  accumLastDataTypeStr=Inherit: Same as product output  roundingMode=Floor  overflowMode=off
  Merge : Merge
  Merge1 : Merge
  Reshape : Reshape  OutputDimensionality=Column vector (2-D)
  Sum1 : Sum  Inputs=+-  SaturateOnIntegerOverflow=on  InputSameDT=on  OutDataTypeStr=Inherit: Same as first input
  Sum4 : Sum  Inputs=+-  SaturateOnIntegerOverflow=on  InputSameDT=on  OutDataTypeStr=Inherit: Same as first input
  Sum5 : Sum  Inputs=2  SaturateOnIntegerOverflow=on  InputSameDT=on  OutDataTypeStr=Inherit: Same as first input
  else : If  IfExpression=u1 > 1  ZeroCross=off
  linear term1 : Product  SaturateOnIntegerOverflow=on  InputSameDT=on  OutDataTypeStr=Inherit: Same as first input
  linear term2 : Product  SaturateOnIntegerOverflow=on  InputSameDT=on  OutDataTypeStr=Inherit: Same as first input
  linear term3 : Product  SaturateOnIntegerOverflow=on  InputSameDT=on  OutDataTypeStr=Inherit: Same as first input
  y : Outport  InitialOutput=0
  wires:
  x/1 -> Check Signal Attributes/1, Inherit Frame Status/2  "X"
  Merge/1 -> linear term1/2  "a"
  linear term1/1 -> Sum5/1
  Merge1/1 -> Sum5/2  "b"
  Sum5/1 -> Sum4/2
  Dot Product2/1 -> linear term3/1, If Action Subsystem/5(In5)
  Matrix Sum1/1 -> If Action Subsystem/4(In4), linear term2/1, linear term2/2
  Maximum/1 -> linear term3/2, If Action Subsystem/2(In2)
  Check Signal Attributes/1 -> Error If Not Floating-Point/1
  Reshape/1 -> Dot Product/2, Matrix Sum2/1, Sum4/1, Constant Ramp/1, Frame Conversion1/1
  Sum4/1 -> Inherit Frame Status/1
  Inherit Frame Status/1 -> y/1
  Constant Ramp/1 -> Dot Product2/2, Matrix Sum1/1, Dot Product2/1, linear term1/1, Dot Product/1, Maximum/1  "ramp"
  else/1 -> If Action Subsystem/Action
  linear term3/1 -> Sum1/1
  linear term2/1 -> Sum1/2
  Dot Product/1 -> If Action Subsystem/1(In1)
  Matrix Sum2/1 -> Frame Conversion/1
  Sum1/1 -> If Action Subsystem1/1(In1), If Action Subsystem/6(In6), else/1
  If Action Subsystem/1(Out1) -> Merge/1
  If Action Subsystem1/2(Out2) -> Merge1/2
  If Action Subsystem/2(Out2) -> Merge1/1
  else/2 -> If Action Subsystem1/Action
  Frame Conversion/1 -> If Action Subsystem/3(In3)
  Frame Conversion1/1 -> If Action Subsystem1/2(In2)
  If Action Subsystem1/1(Out1) -> Merge/2
  Error If Not Floating-Point/1 -> Reshape/1

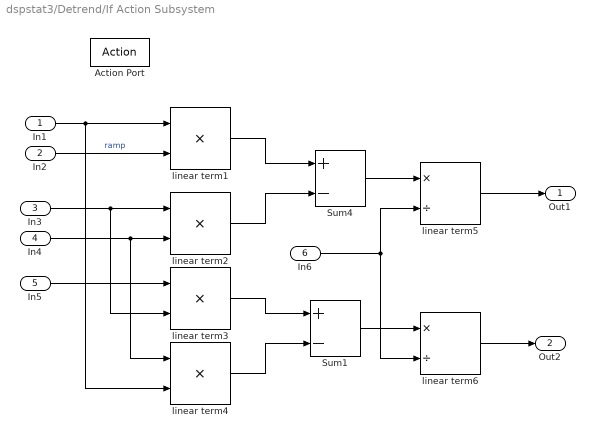
== system dspstat3/Detrend/If Action Subsystem ==
  In1 : Inport
  In2 : Inport  Port=2
  In3 : Inport  Port=3
  In4 : Inport  Port=4
  In5 : Inport  Port=5
  In6 : Inport  Port=6
  Action Port : ActionPort  PropagateVarSize=During execution
  Sum1 : Sum  Inputs=+-  SaturateOnIntegerOverflow=on  InputSameDT=on  OutDataTypeStr=Inherit: Same as first input
  Sum4 : Sum  Inputs=+-  SaturateOnIntegerOverflow=on  InputSameDT=on  OutDataTypeStr=Inherit: Same as first input
  linear term{1..4} (4 alike) : Product  SaturateOnIntegerOverflow=on  InputSameDT=on  OutDataTypeStr=Inherit: Same as first input
  linear term5 : Product  Inputs=*/  SaturateOnIntegerOverflow=on  InputSameDT=on  OutDataTypeStr=Inherit: Same as first input
  linear term6 : Product  Inputs=*/  SaturateOnIntegerOverflow=on  InputSameDT=on  OutDataTypeStr=Inherit: Same as first input
  Out1 : Outport
  Out2 : Outport  Port=2
  wires:
  In1/1 -> linear term1/1, linear term4/2
  In2/1 -> linear term1/2  "ramp"
  In3/1 -> linear term2/1, linear term3/2
  In4/1 -> linear term2/2, linear term4/1
  linear term1/1 -> Sum4/1
  linear term2/1 -> Sum4/2
  linear term3/1 -> Sum1/1
  linear term4/1 -> Sum1/2
  In6/1 -> linear term5/2, linear term6/2
  Sum4/1 -> linear term5/1
  Sum1/1 -> linear term6/1
  In5/1 -> linear term3/1
  linear term5/1 -> Out1/1
  linear term6/1 -> Out2/1

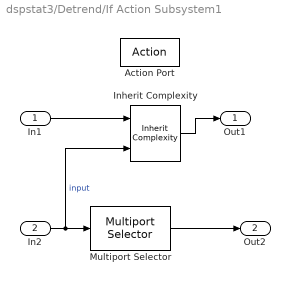
== system dspstat3/Detrend/If Action Subsystem1 ==
  In1 : Inport
  In2 : Inport  Port=2
  Action Port : ActionPort  PropagateVarSize=During execution
  Inherit Complexity : dspsigattribs/Inherit Complexity
  Multiport Selector : dspindex/Multiport Selector  rowsOrCols=Rows  idxCellArray=1  idxErrMode=Clip Index
  Out1 : Outport
  Out2 : Outport  Port=2
  wires:
  In2/1 -> Multiport Selector/1, Inherit Complexity/2  "input"
  Multiport Selector/1 -> Out2/1
  In1/1 -> Inherit Complexity/1
  Inherit Complexity/1 -> Out1/1
